simulink model "nominal_system"  (R2018a)
settings: Solver=ode8  StartTime=0.0  StopTime=10  FixedStep=.001  MaxStep=0.01  MinStep=.001  RelTol=1e-3
values from neighbouring files (symbols this model uses):
  a = 1.4    [Codefile.m]
  alpha1 = 0    [Codefile.m]
  Ap1 = 0    [Codefile.m]
  b = 1.7    [Codefile.m]
  beta1 = 0    [Codefile.m]
  c = 1.5    [Codefile.m]    (also in Quater_car.m = [700 1500 3000])
  Csfl = 1000    [Codefile.m]
  Csfr = 1000    [Codefile.m]
  Csrl = 1100    [Codefile.m]
  Csrr = 1100    [Codefile.m]
  d = 1.5    [Codefile.m]
  delay = (a+b)/v    (= 0.3875)    [Codefile.m]
  G = [ 0          0      0           0, ... (first row only)    [Codefile.m]
  gama1 = 0    [Codefile.m]
  Ixx = 460    [Codefile.m]
  Iyy = 2160    [Codefile.m]
  Ksfl = 35000    [Codefile.m]
  Ksfr = 35000    [Codefile.m]
  Ksrl = 38000    [Codefile.m]
  Ksrr = 38000    [Codefile.m]
  Kufl = 190000    [Codefile.m]
  Kufr = 190000    [Codefile.m]
  Kurl = 190000    [Codefile.m]
  Kurr = 190000    [Codefile.m]
  M = 1500    [Codefile.m]    (also in Quater_car.m = 117; half_car.m = 117)
  m = 59    [Codefile.m]    (also in Quater_car.m = 30)
  Ps1 = 0    [Codefile.m]
  tau1 = 1    [Codefile.m]
settings Model: Creator=Student  LastModifiedBy=Student
settings SolverCC: InitialStep=.001

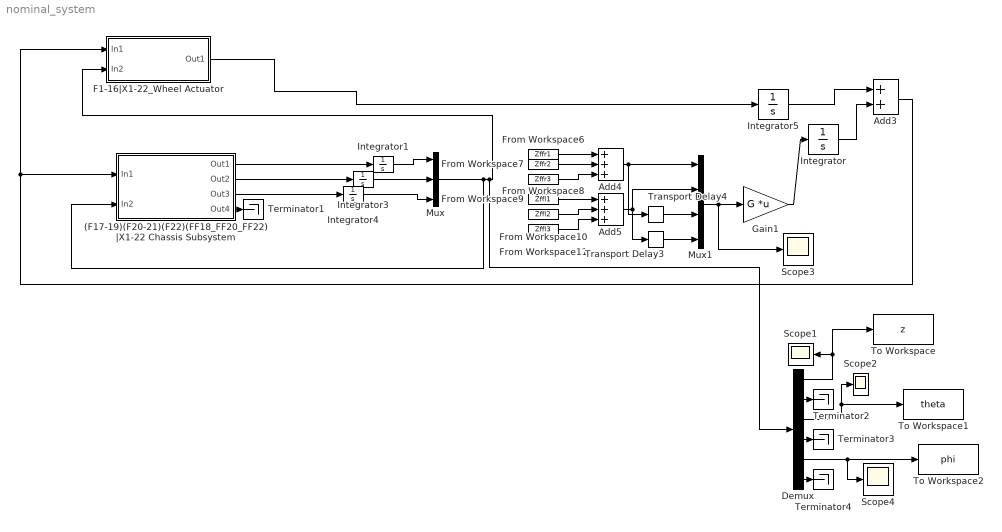
== system nominal_system ==
  "(F17-19)(F20-21)(F22)(FF18_FF20_FF22) |X1-22 Chassis Subsystem " : Subsystem  TreatAsAtomicUnit=on
  Add3 : Sum  Inputs=2
  Add4 : Sum  Inputs=3
  Add5 : Sum  Inputs=3
  Demux : Demux  Outputs=6
  "F1-16|X1-22_Wheel Actuator " : Subsystem  TreatAsAtomicUnit=on
  From Workspace10 : FromWorkspace  VariableName=Zffl2  SampleTime=0  Interpolate=off  OutputAfterFinalValue=Setting to zero
  From Workspace11 : FromWorkspace  VariableName=Zffl3  SampleTime=0  Interpolate=off  OutputAfterFinalValue=Setting to zero
  From Workspace6 : FromWorkspace  VariableName=Zffr1  SampleTime=0  Interpolate=off  OutputAfterFinalValue=Setting to zero
  From Workspace7 : FromWorkspace  VariableName=Zffr2  SampleTime=0  Interpolate=off  OutputAfterFinalValue=Setting to zero
  From Workspace8 : FromWorkspace  VariableName=Zffr3  SampleTime=0  Interpolate=off  OutputAfterFinalValue=Setting to zero
  From Workspace9 : FromWorkspace  VariableName=Zffl1  SampleTime=0  Interpolate=off  OutputAfterFinalValue=Setting to zero
  Gain1 : Gain  Gain=G  Multiplication=Matrix(K*u)
  Integrator{,1,3..5} (5 alike) : Integrator  AbsoluteTolerance=1e-4
  Mux : Mux  Inputs=3
  Mux1 : Mux
  Scope{1..4} (4 alike) : Scope
  Terminator{1..4} (4 alike) : Terminator
  To Workspace : ToWorkspace  VariableName=z  SaveFormat=Timeseries  SampleTime=-1
  To Workspace1 : ToWorkspace  VariableName=theta  SaveFormat=Timeseries  SampleTime=-1
  To Workspace2 : ToWorkspace  VariableName=phi  SaveFormat=Timeseries  SampleTime=-1
  Transport Delay3 : TransportDelay  DelayTime=delay
  Transport Delay4 : TransportDelay  DelayTime=delay
  wires:
  Demux/6 -> Terminator4/1
  Integrator4/1 -> Mux/3
  Demux/2 -> Terminator2/1
  Demux/3 -> Scope2/1, To Workspace1/1
  Integrator/1 -> Add3/2
  Integrator1/1 -> Mux/1
  Integrator3/1 -> Mux/2
  Integrator5/1 -> Add3/1
  "F1-16|X1-22_Wheel Actuator "/1(Out1) -> Integrator5/1
  "(F17-19)(F20-21)(F22)(FF18_FF20_FF22) |X1-22 Chassis Subsystem "/3(Out3) -> Integrator4/1
  Add3/1 -> "F1-16|X1-22_Wheel Actuator "/1(In1), "(F17-19)(F20-21)(F22)(FF18_FF20_FF22) |X1-22 Chassis Subsystem "/1(In1)
  Mux/1 -> "(F17-19)(F20-21)(F22)(FF18_FF20_FF22) |X1-22 Chassis Subsystem "/2(In2), Demux/1, "F1-16|X1-22_Wheel Actuator "/2(In2)
  Demux/4 -> Terminator3/1
  "(F17-19)(F20-21)(F22)(FF18_FF20_FF22) |X1-22 Chassis Subsystem "/2(Out2) -> Integrator3/1
  Gain1/1 -> Integrator/1
  "(F17-19)(F20-21)(F22)(FF18_FF20_FF22) |X1-22 Chassis Subsystem "/1(Out1) -> Integrator1/1
  Demux/5 -> To Workspace2/1, Scope4/1
  "(F17-19)(F20-21)(F22)(FF18_FF20_FF22) |X1-22 Chassis Subsystem "/4(Out4) -> Terminator1/1
  From Workspace7/1 -> Add4/2
  From Workspace10/1 -> Add5/2
  From Workspace11/1 -> Add5/3
  From Workspace9/1 -> Add5/1
  Add5/1 -> Mux1/2, Transport Delay3/1
  From Workspace6/1 -> Add4/1
  From Workspace8/1 -> Add4/3
  Mux1/1 -> Scope3/1, Gain1/1
  Add4/1 -> Mux1/1, Transport Delay4/1
  Transport Delay4/1 -> Mux1/3
  Transport Delay3/1 -> Mux1/4
  Demux/1 -> To Workspace/1, Scope1/1

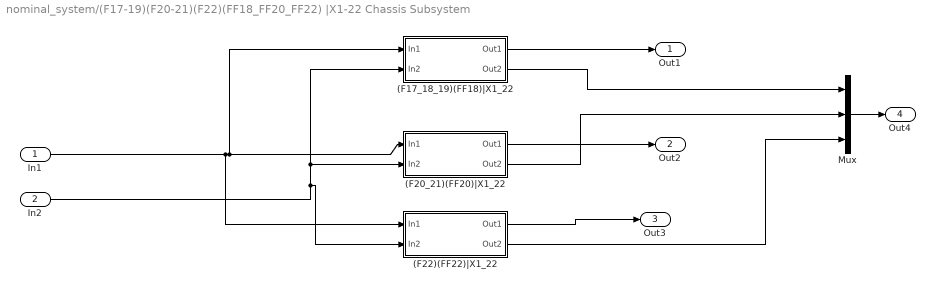
== system nominal_system/(F17-19)(F20-21)(F22)(FF18_FF20_FF22) |X1-22 Chassis Subsystem  ==
  In1 : Inport
  In2 : Inport  Port=2
  (F17_18_19)(FF18)|X1_22 : Subsystem  TreatAsAtomicUnit=on
  "(F20_21)(FF20)|X1_22 " : Subsystem  TreatAsAtomicUnit=on
  (F22)(FF22)|X1_22 : Subsystem  TreatAsAtomicUnit=on
  Mux : Mux  Inputs=3
  Out1 : Outport
  Out2 : Outport  Port=2
  Out3 : Outport  Port=3
  Out4 : Outport  Port=4
  wires:
  In1/1 -> (F17_18_19)(FF18)|X1_22/1(In1), "(F20_21)(FF20)|X1_22 "/1(In1), (F22)(FF22)|X1_22/1(In1)
  (F22)(FF22)|X1_22/1(Out1) -> Out3/1
  "(F20_21)(FF20)|X1_22 "/1(Out1) -> Out2/1
  (F17_18_19)(FF18)|X1_22/1(Out1) -> Out1/1
  (F17_18_19)(FF18)|X1_22/2(Out2) -> Mux/1
  "(F20_21)(FF20)|X1_22 "/2(Out2) -> Mux/2
  (F22)(FF22)|X1_22/2(Out2) -> Mux/3
  Mux/1 -> Out4/1
  In2/1 -> (F22)(FF22)|X1_22/2(In2), "(F20_21)(FF20)|X1_22 "/2(In2), (F17_18_19)(FF18)|X1_22/2(In2)

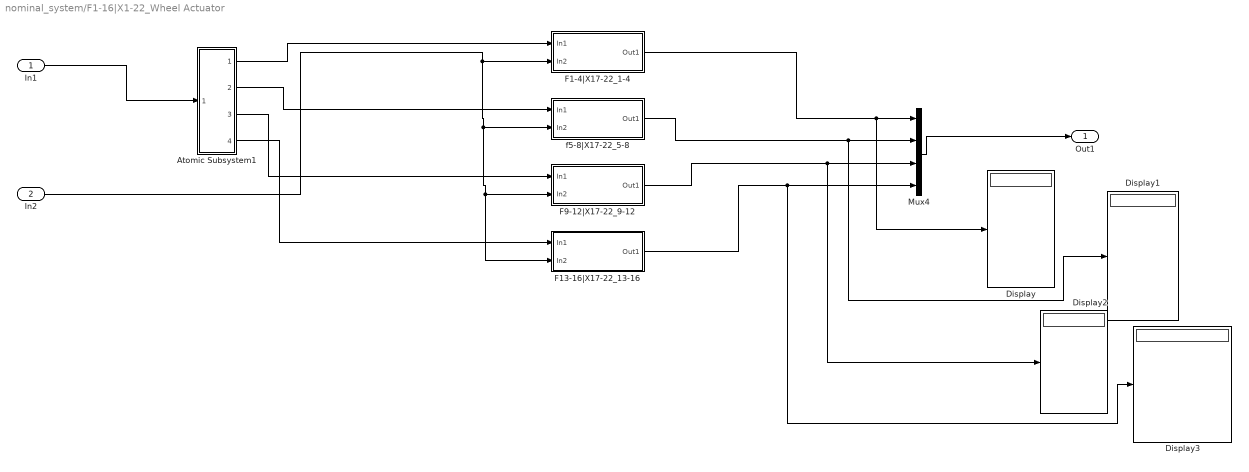
== system nominal_system/F1-16|X1-22_Wheel Actuator  ==
  In1 : Inport
  In2 : Inport  Port=2
  Atomic Subsystem1 : Subsystem  TreatAsAtomicUnit=on
  Display{,1..3} (4 alike) : Display
  F1-4|X17-22_1-4 : Subsystem  TreatAsAtomicUnit=on
  F13-16|X17-22_13-16 : Subsystem  TreatAsAtomicUnit=on
  F9-12|X17-22_9-12 : Subsystem  TreatAsAtomicUnit=on
  Mux4 : Mux
  f5-8|X17-22_5-8 : Subsystem  TreatAsAtomicUnit=on
  Out1 : Outport
  wires:
  In1/1 -> Atomic Subsystem1/1(In1)
  Mux4/1 -> Out1/1
  Atomic Subsystem1/1(Out1) -> F1-4|X17-22_1-4/1(In1)
  Atomic Subsystem1/2(Out2) -> f5-8|X17-22_5-8/1(In1)
  Atomic Subsystem1/3(Out3) -> F9-12|X17-22_9-12/1(In1)
  Atomic Subsystem1/4(Out4) -> F13-16|X17-22_13-16/1(In1)
  In2/1 -> F13-16|X17-22_13-16/2(In2), F9-12|X17-22_9-12/2(In2), f5-8|X17-22_5-8/2(In2), F1-4|X17-22_1-4/2(In2)
  F1-4|X17-22_1-4/1(Out1) -> Display/1, Mux4/1
  f5-8|X17-22_5-8/1(Out1) -> Display1/1, Mux4/2
  F9-12|X17-22_9-12/1(Out1) -> Display2/1, Mux4/3
  F13-16|X17-22_13-16/1(Out1) -> Display3/1, Mux4/4

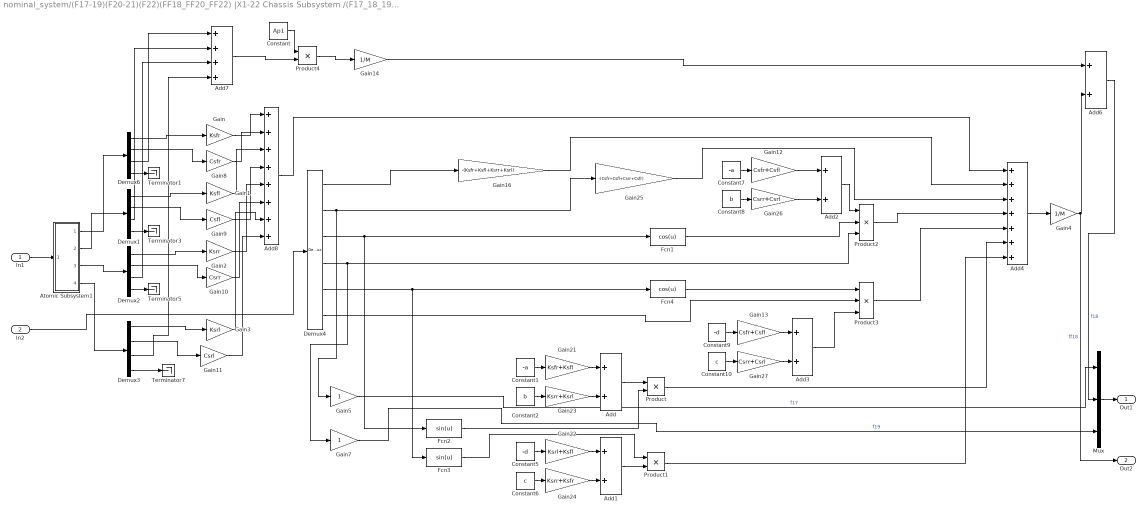
== system nominal_system/(F17-19)(F20-21)(F22)(FF18_FF20_FF22) |X1-22 Chassis Subsystem /(F17_18_19)(FF18)|X1_22 ==
  In1 : Inport
  In2 : Inport  Port=2
  Add{,1..3,6} (5 alike) : Sum
  Add4 : Sum  Inputs=+++++++
  Add7 : Sum  Inputs=++++
  Add8 : Sum  Inputs=++++++++
  Atomic Subsystem1 : Subsystem  TreatAsAtomicUnit=on
  Constant : Constant  Value=Ap1
  Constant1 : Constant  Value=-a
  Constant10 : Constant  Value=c
  Constant2 : Constant  Value=b
  Constant5 : Constant  Value=-d
  Constant6 : Constant  Value=c
  Constant7 : Constant  Value=-a
  Constant8 : Constant  Value=b
  Constant9 : Constant  Value=-d
  Demux{1..3,6} (4 alike) : Demux
  Demux4 : Demux  Outputs=6
  Fcn1 : Fcn  Expr=cos(u)
  Fcn2 : Fcn  Expr=sin(u)
  Fcn3 : Fcn  Expr=sin(u)
  Fcn4 : Fcn  Expr=cos(u)
  Gain : Gain  Gain=Ksfr
  Gain1 : Gain  Gain=Ksfl
  Gain10 : Gain  Gain=Csrr
  Gain11 : Gain  Gain=Csrl
  Gain12 : Gain  Gain=Csfr+Csfl
  Gain13 : Gain  Gain=Csfr+Csfl
  Gain14 : Gain  Gain=1/M
  Gain16 : Gain  Gain=-(Ksfr+Ksfl+Ksrr+Ksrl)
  Gain2 : Gain  Gain=Ksrr
  Gain21 : Gain  Gain=Ksfr+Ksfl
  Gain22 : Gain  Gain=Ksrl+Ksfl
  Gain23 : Gain  Gain=Ksrr+Ksrl
  Gain24 : Gain  Gain=Ksrr+Ksfr
  Gain25 : Gain  Gain=-(Csfr+Csfl+Csrr+Csfr)
  Gain26 : Gain  Gain=Csrr+Csrl
  Gain27 : Gain  Gain=Csrr+Csrl
  Gain3 : Gain  Gain=Ksrl
  Gain4 : Gain  Gain=1/M
  Gain5 : Gain
  Gain7 : Gain
  Gain8 : Gain  Gain=Csfr
  Gain9 : Gain  Gain=Csfl
  Mux : Mux  Inputs=3
  Product : Product
  Product1 : Product
  Product2 : Product  Inputs=3
  Product3 : Product  Inputs=3
  Product4 : Product
  Terminator{1,3,5,7} (4 alike) : Terminator
  Out1 : Outport
  Out2 : Outport  Port=2
  wires:
  Demux6/1 -> Gain/1
  Demux1/1 -> Gain1/1
  Demux2/1 -> Gain2/1
  Demux3/1 -> Gain3/1
  Demux4/1 -> Gain16/1
  Demux4/3 -> Fcn2/1, Fcn1/1
  Gain21/1 -> Add/1
  Constant1/1 -> Gain21/1
  Gain23/1 -> Add/2
  Constant2/1 -> Gain23/1
  Add/1 -> Product/1
  Fcn2/1 -> Product/2
  Demux4/5 -> Fcn3/1, Fcn4/1
  Gain22/1 -> Add1/1
  Gain24/1 -> Add1/2
  Constant5/1 -> Gain22/1
  Constant6/1 -> Gain24/1
  Add1/1 -> Product1/2
  Fcn3/1 -> Product1/1
  Demux4/2 -> Gain5/1, Gain25/1
  Demux4/4 -> Gain7/1, Product2/3
  Fcn1/1 -> Product2/2
  Gain12/1 -> Add2/1
  Constant7/1 -> Gain12/1
  Gain26/1 -> Add2/2
  Constant8/1 -> Gain26/1
  Add2/1 -> Product2/1
  Gain13/1 -> Add3/1
  Constant9/1 -> Gain13/1
  Gain27/1 -> Add3/2
  Constant10/1 -> Gain27/1
  Fcn4/1 -> Product3/1
  Demux4/6 -> Product3/2
  Add3/1 -> Product3/3
  Product/1 -> Add4/6
  Product1/1 -> Add4/7
  Add4/1 -> Gain4/1
  Gain14/1 -> Add6/1
  Gain4/1 -> Out2/1, Add6/2  "ff18"
  Add6/1 -> Mux/2  "f18"
  Gain5/1 -> Mux/1  "f17"
  Gain7/1 -> Mux/3  "f19"
  Demux6/2 -> Gain8/1
  Demux1/2 -> Gain9/1
  Demux2/2 -> Gain10/1
  Demux3/2 -> Gain11/1
  Gain/1 -> Add8/1
  Gain8/1 -> Add8/2
  Gain1/1 -> Add8/3
  Gain9/1 -> Add8/4
  Gain2/1 -> Add8/5
  Gain10/1 -> Add8/6
  Gain3/1 -> Add8/7
  Gain11/1 -> Add8/8
  Product3/1 -> Add4/5
  Product2/1 -> Add4/4
  Gain25/1 -> Add4/3
  Gain16/1 -> Add4/2
  Add8/1 -> Add4/1
  Demux6/3 -> Add7/1
  Demux6/4 -> Terminator1/1
  Demux1/3 -> Add7/2
  Demux1/4 -> Terminator3/1
  Demux2/3 -> Add7/3
  Demux2/4 -> Terminator5/1
  Demux3/3 -> Add7/4
  Demux3/4 -> Terminator7/1
  Mux/1 -> Out1/1
  Add7/1 -> Product4/2
  Constant/1 -> Product4/1
  Product4/1 -> Gain14/1
  In1/1 -> Atomic Subsystem1/1(In1)
  Atomic Subsystem1/1(Out1) -> Demux6/1
  Atomic Subsystem1/2(Out2) -> Demux1/1
  Atomic Subsystem1/3(Out3) -> Demux2/1
  Atomic Subsystem1/4(Out4) -> Demux3/1
  In2/1 -> Demux4/1

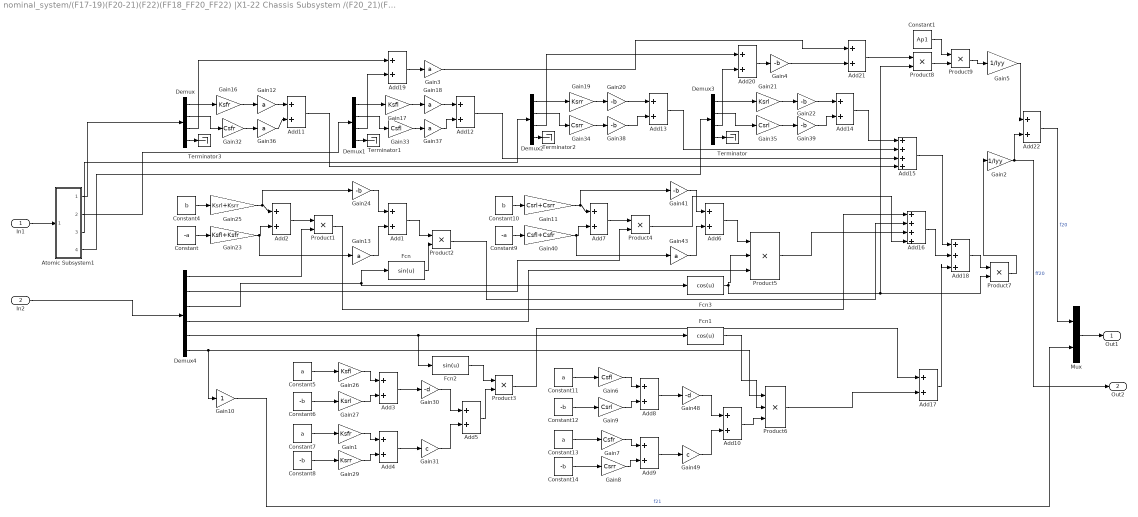
== system nominal_system/(F17-19)(F20-21)(F22)(FF18_FF20_FF22) |X1-22 Chassis Subsystem /(F20_21)(FF20)|X1_22  ==
  In1 : Inport
  In2 : Inport  Port=2
  Add{1..14,17,19..22} (19 alike) : Sum
  Add15 : Sum  Inputs=++++
  Add16 : Sum  Inputs=++++
  Add18 : Sum  Inputs=+++
  Atomic Subsystem1 : Subsystem  TreatAsAtomicUnit=on
  Constant : Constant  Value=-a
  Constant1 : Constant  Value=Ap1
  Constant10 : Constant  Value=b
  Constant{5,7,11,13} (4 alike) : Constant  Value=a
  Constant{6,8,12,14} (4 alike) : Constant  Value=-b
  Constant4 : Constant  Value=b
  Constant9 : Constant  Value=-a
  Demux{,1..3} (4 alike) : Demux
  Demux4 : Demux  Outputs=6
  Fcn : Fcn  Expr=sin(u)
  Fcn1 : Fcn  Expr=cos(u)
  Fcn2 : Fcn  Expr=sin(u)
  Fcn3 : Fcn  Expr=cos(u)
  Gain1 : Gain  Gain=Ksfr
  Gain10 : Gain
  Gain11 : Gain  Gain=Csrl+Csrr
  Gain{3,12..13,18,36..37,43} (7 alike) : Gain  Gain=a
  Gain16 : Gain  Gain=Ksfr
  Gain17 : Gain  Gain=Ksfl
  Gain19 : Gain  Gain=Ksrr
  Gain2 : Gain  Gain=1/Iyy
  Gain{4,20,22,24,38..39,41} (7 alike) : Gain  Gain=-b
  Gain21 : Gain  Gain=Ksrl
  Gain23 : Gain  Gain=Ksfl+Ksfr
  Gain25 : Gain  Gain=Ksrl+Ksrr
  Gain26 : Gain  Gain=Ksfl
  Gain27 : Gain  Gain=Ksrl
  Gain29 : Gain  Gain=Ksrr
  Gain30 : Gain  Gain=-d
  Gain31 : Gain  Gain=c
  Gain32 : Gain  Gain=Csfr
  Gain33 : Gain  Gain=Csfl
  Gain34 : Gain  Gain=Csrr
  Gain35 : Gain  Gain=Csrl
  Gain40 : Gain  Gain=Csfl+Csfr
  Gain48 : Gain  Gain=-d
  Gain49 : Gain  Gain=c
  Gain5 : Gain  Gain=1/Iyy
  Gain6 : Gain  Gain=Csfl
  Gain7 : Gain  Gain=Csfr
  Gain8 : Gain  Gain=Csrr
  Gain9 : Gain  Gain=Csrl
  Mux : Mux  Inputs=2
  Product{1..4,7..9} (7 alike) : Product
  Product5 : Product  Inputs=3
  Product6 : Product  Inputs=3
  Terminator{,1..3} (4 alike) : Terminator
  Out1 : Outport
  Out2 : Outport  Port=2
  wires:
  Demux/1 -> Gain16/1
  Gain16/1 -> Gain12/1
  Demux1/1 -> Gain17/1
  Gain17/1 -> Gain18/1
  Demux2/1 -> Gain19/1
  Gain19/1 -> Gain20/1
  Demux3/1 -> Gain21/1
  Gain21/1 -> Gain22/1
  Constant/1 -> Gain23/1
  Constant4/1 -> Gain25/1
  Gain23/1 -> Gain13/1, Add2/2
  Gain25/1 -> Gain24/1, Add2/1
  Add2/1 -> Product1/1
  Demux4/1 -> Product1/2
  Gain24/1 -> Add1/1
  Gain13/1 -> Add1/2
  Constant5/1 -> Gain26/1
  Constant6/1 -> Gain27/1
  Gain26/1 -> Add3/1
  Gain27/1 -> Add3/2
  Constant8/1 -> Gain29/1
  Constant7/1 -> Gain1/1
  Gain1/1 -> Add4/1
  Gain29/1 -> Add4/2
  Add3/1 -> Gain30/1
  Add4/1 -> Gain31/1
  Demux4/3 -> Fcn3/1, Fcn/1
  Add1/1 -> Product2/1
  Fcn/1 -> Product2/2
  Demux4/5 -> Fcn1/1, Fcn2/1
  Gain30/1 -> Add5/1
  Gain31/1 -> Add5/2
  Add5/1 -> Product3/2
  Fcn2/1 -> Product3/1
  Demux/2 -> Gain32/1
  Demux1/2 -> Gain33/1
  Demux2/2 -> Gain34/1
  Demux3/2 -> Gain35/1
  Gain32/1 -> Gain36/1
  Gain33/1 -> Gain37/1
  Gain34/1 -> Gain38/1
  Gain35/1 -> Gain39/1
  Constant10/1 -> Gain11/1
  Gain40/1 -> Gain43/1, Add7/2
  Gain11/1 -> Add7/1, Gain41/1
  Add7/1 -> Product4/1
  Demux4/2 -> Product4/2
  Gain41/1 -> Add6/1
  Gain43/1 -> Add6/2
  Add6/1 -> Product5/1
  Constant9/1 -> Gain40/1
  Fcn3/1 -> Product5/2, Product8/2, Product7/2
  Demux4/4 -> Product5/3
  Constant11/1 -> Gain6/1
  Constant12/1 -> Gain9/1
  Gain6/1 -> Add8/1
  Gain9/1 -> Add8/2
  Constant14/1 -> Gain8/1
  Constant13/1 -> Gain7/1
  Gain7/1 -> Add9/1
  Add8/1 -> Gain48/1
  Add9/1 -> Gain49/1
  Gain48/1 -> Add10/1
  Gain49/1 -> Add10/2
  Add10/1 -> Product6/3
  Fcn1/1 -> Product6/2
  Gain8/1 -> Add9/2
  Demux4/6 -> Gain10/1, Product6/1
  Gain12/1 -> Add11/1
  Gain36/1 -> Add11/2
  Gain18/1 -> Add12/1
  Gain37/1 -> Add12/2
  Gain20/1 -> Add13/1
  Gain38/1 -> Add13/2
  Gain22/1 -> Add14/1
  Gain39/1 -> Add14/2
  Add14/1 -> Add15/1
  Add13/1 -> Add15/2
  Add12/1 -> Add15/3
  Add11/1 -> Add15/4
  Product1/1 -> Add16/1
  Product2/1 -> Add16/2
  Product5/1 -> Add16/3
  Product4/1 -> Add16/4
  Product3/1 -> Add17/1
  Product6/1 -> Add17/2
  Add15/1 -> Add18/1
  Add17/1 -> Add18/3
  Add16/1 -> Add18/2
  Add18/1 -> Product7/1
  Product7/1 -> Gain2/1
  Demux/3 -> Add19/1
  Demux1/3 -> Add19/2
  Add19/1 -> Gain3/1
  Demux2/3 -> Add20/1
  Demux3/3 -> Add20/2
  Add20/1 -> Gain4/1
  Gain4/1 -> Add21/2
  Gain3/1 -> Add21/1
  Add21/1 -> Product8/1
  Gain5/1 -> Add22/1
  Gain2/1 -> Out2/1, Add22/2  "ff20"
  Gain10/1 -> Mux/2  "f21"
  Add22/1 -> Mux/1  "f20"
  Demux1/4 -> Terminator1/1
  Demux2/4 -> Terminator2/1
  Demux3/4 -> Terminator/1
  Demux/4 -> Terminator3/1
  In2/1 -> Demux4/1
  Atomic Subsystem1/1(Out1) -> Demux/1
  Atomic Subsystem1/2(Out2) -> Demux1/1
  Atomic Subsystem1/3(Out3) -> Demux2/1
  Atomic Subsystem1/4(Out4) -> Demux3/1
  Mux/1 -> Out1/1
  Product8/1 -> Product9/2
  Product9/1 -> Gain5/1
  Constant1/1 -> Product9/1
  In1/1 -> Atomic Subsystem1/1(In1)

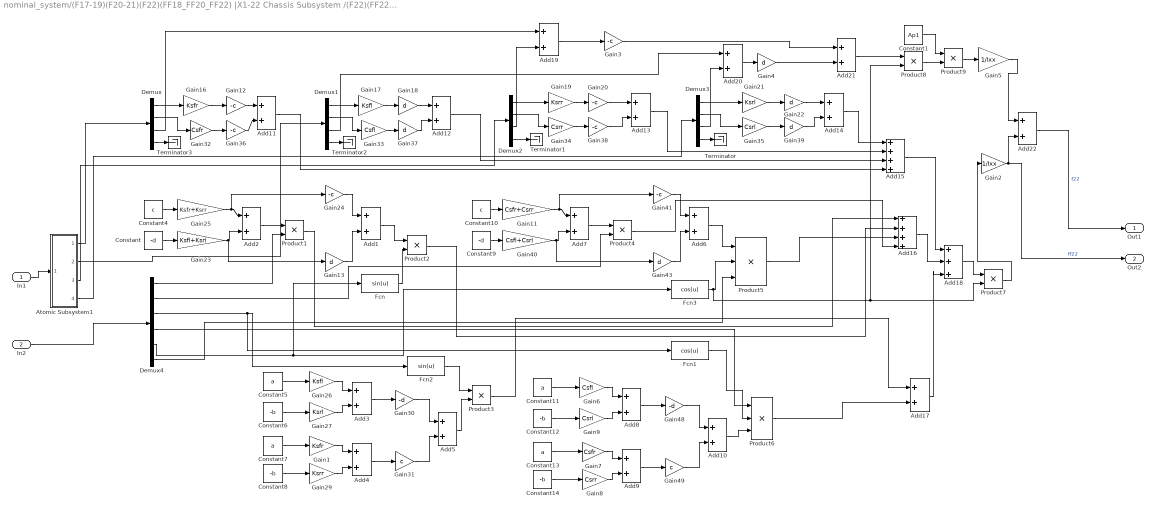
== system nominal_system/(F17-19)(F20-21)(F22)(FF18_FF20_FF22) |X1-22 Chassis Subsystem /(F22)(FF22)|X1_22 ==
  In1 : Inport
  In2 : Inport  Port=2
  Add{1..14,17,19..22} (19 alike) : Sum
  Add15 : Sum  Inputs=++++
  Add16 : Sum  Inputs=++++
  Add18 : Sum  Inputs=+++
  Atomic Subsystem1 : Subsystem  TreatAsAtomicUnit=on
  Constant : Constant  Value=-d
  Constant1 : Constant  Value=Ap1
  Constant10 : Constant  Value=c
  Constant{5,7,11,13} (4 alike) : Constant  Value=a
  Constant{6,8,12,14} (4 alike) : Constant  Value=-b
  Constant4 : Constant  Value=c
  Constant9 : Constant  Value=-d
  Demux{,1..3} (4 alike) : Demux
  Demux4 : Demux  Outputs=6
  Fcn : Fcn  Expr=sin(u)
  Fcn1 : Fcn  Expr=cos(u)
  Fcn2 : Fcn  Expr=sin(u)
  Fcn3 : Fcn  Expr=cos(u)
  Gain1 : Gain  Gain=Ksfr
  Gain11 : Gain  Gain=Csfr+Csrr
  Gain{3,12,20,24,36,38,41} (7 alike) : Gain  Gain=-c
  Gain{4,13,18,22,37,39,43} (7 alike) : Gain  Gain=d
  Gain16 : Gain  Gain=Ksfr
  Gain17 : Gain  Gain=Ksfl
  Gain19 : Gain  Gain=Ksrr
  Gain2 : Gain  Gain=1/Ixx
  Gain21 : Gain  Gain=Ksrl
  Gain23 : Gain  Gain=Ksfl+Ksrl
  Gain25 : Gain  Gain=Ksfr+Ksrr
  Gain26 : Gain  Gain=Ksfl
  Gain27 : Gain  Gain=Ksrl
  Gain29 : Gain  Gain=Ksrr
  Gain30 : Gain  Gain=-d
  Gain31 : Gain  Gain=c
  Gain32 : Gain  Gain=Csfr
  Gain33 : Gain  Gain=Csfl
  Gain34 : Gain  Gain=Csrr
  Gain35 : Gain  Gain=Csrl
  Gain40 : Gain  Gain=Csfl+Csrl
  Gain48 : Gain  Gain=-d
  Gain49 : Gain  Gain=c
  Gain5 : Gain  Gain=1/Ixx
  Gain6 : Gain  Gain=Csfl
  Gain7 : Gain  Gain=Csfr
  Gain8 : Gain  Gain=Csrr
  Gain9 : Gain  Gain=Csrl
  Product{1..4,7..9} (7 alike) : Product
  Product5 : Product  Inputs=3
  Product6 : Product  Inputs=3
  Terminator{,1..3} (4 alike) : Terminator
  Out1 : Outport
  Out2 : Outport  Port=2
  wires:
  Demux/1 -> Gain16/1
  Gain16/1 -> Gain12/1
  Demux1/1 -> Gain17/1
  Gain17/1 -> Gain18/1
  Demux2/1 -> Gain19/1
  Gain19/1 -> Gain20/1
  Demux3/1 -> Gain21/1
  Gain21/1 -> Gain22/1
  Constant/1 -> Gain23/1
  Constant4/1 -> Gain25/1
  Gain23/1 -> Gain13/1, Add2/2
  Gain25/1 -> Gain24/1, Add2/1
  Add2/1 -> Product1/1
  Demux4/1 -> Product1/2
  Gain24/1 -> Add1/1
  Gain13/1 -> Add1/2
  Constant5/1 -> Gain26/1
  Constant6/1 -> Gain27/1
  Gain26/1 -> Add3/1
  Gain27/1 -> Add3/2
  Constant8/1 -> Gain29/1
  Constant7/1 -> Gain1/1
  Gain1/1 -> Add4/1
  Gain29/1 -> Add4/2
  Add3/1 -> Gain30/1
  Add4/1 -> Gain31/1
  Demux4/3 -> Fcn1/1, Fcn2/1
  Add1/1 -> Product2/1
  Fcn/1 -> Product2/2
  Demux4/5 -> Fcn/1, Fcn3/1
  Gain30/1 -> Add5/1
  Gain31/1 -> Add5/2
  Add5/1 -> Product3/2
  Fcn2/1 -> Product3/1
  Demux/2 -> Gain32/1
  Demux1/2 -> Gain33/1
  Demux2/2 -> Gain34/1
  Demux3/2 -> Gain35/1
  Gain32/1 -> Gain36/1
  Gain33/1 -> Gain37/1
  Gain34/1 -> Gain38/1
  Gain35/1 -> Gain39/1
  Constant10/1 -> Gain11/1
  Gain40/1 -> Gain43/1, Add7/2
  Gain11/1 -> Add7/1, Gain41/1
  Add7/1 -> Product4/1
  Demux4/2 -> Product4/2
  Gain41/1 -> Add6/1
  Gain43/1 -> Add6/2
  Add6/1 -> Product5/1
  Constant9/1 -> Gain40/1
  Fcn3/1 -> Product8/2, Product7/2, Product5/2
  Constant11/1 -> Gain6/1
  Constant12/1 -> Gain9/1
  Gain6/1 -> Add8/1
  Gain9/1 -> Add8/2
  Constant14/1 -> Gain8/1
  Constant13/1 -> Gain7/1
  Gain7/1 -> Add9/1
  Add8/1 -> Gain48/1
  Add9/1 -> Gain49/1
  Gain48/1 -> Add10/1
  Gain49/1 -> Add10/2
  Add10/1 -> Product6/3
  Fcn1/1 -> Product6/2
  Gain8/1 -> Add9/2
  Demux4/6 -> Product5/3
  Gain12/1 -> Add11/1
  Gain36/1 -> Add11/2
  Gain18/1 -> Add12/1
  Gain37/1 -> Add12/2
  Gain20/1 -> Add13/1
  Gain38/1 -> Add13/2
  Gain22/1 -> Add14/1
  Gain39/1 -> Add14/2
  Add14/1 -> Add15/1
  Add13/1 -> Add15/2
  Add12/1 -> Add15/3
  Add11/1 -> Add15/4
  Product1/1 -> Add16/1
  Product2/1 -> Add16/2
  Product5/1 -> Add16/3
  Product4/1 -> Add16/4
  Product3/1 -> Add17/1
  Product6/1 -> Add17/2
  Add15/1 -> Add18/1
  Add17/1 -> Add18/3
  Add16/1 -> Add18/2
  Add18/1 -> Product7/1
  Product7/1 -> Gain2/1
  Demux/3 -> Add19/1
  Add19/1 -> Gain3/1
  Add20/1 -> Gain4/1
  Gain4/1 -> Add21/2
  Gain3/1 -> Add21/1
  Add21/1 -> Product8/1
  Gain5/1 -> Add22/1
  Gain2/1 -> Out2/1, Add22/2  "ff22"
  Add22/1 -> Out1/1  "f22"
  Demux4/4 -> Product6/1
  Demux2/3 -> Add19/2
  Demux1/3 -> Add20/1
  Demux3/3 -> Add20/2
  In2/1 -> Demux4/1
  Atomic Subsystem1/1(Out1) -> Demux/1
  Atomic Subsystem1/2(Out2) -> Demux1/1
  Atomic Subsystem1/3(Out3) -> Demux2/1
  Atomic Subsystem1/4(Out4) -> Demux3/1
  Demux3/4 -> Terminator/1
  Demux2/4 -> Terminator1/1
  Demux1/4 -> Terminator2/1
  Demux/4 -> Terminator3/1
  In1/1 -> Atomic Subsystem1/1(In1)
  Product9/1 -> Gain5/1
  Product8/1 -> Product9/2
  Constant1/1 -> Product9/1

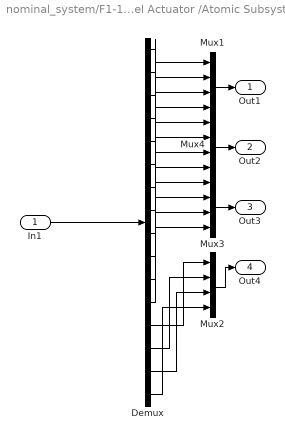
== system nominal_system/F1-16|X1-22_Wheel Actuator /Atomic Subsystem1 ==
  In1 : Inport
  Demux : Demux  Outputs=16
  Mux{1..4} (4 alike) : Mux
  Out1 : Outport
  Out2 : Outport  Port=2
  Out3 : Outport  Port=3
  Out4 : Outport  Port=4
  wires:
  In1/1 -> Demux/1
  Demux/16 -> Mux2/4
  Demux/15 -> Mux2/3
  Demux/14 -> Mux2/2
  Demux/13 -> Mux2/1
  Demux/12 -> Mux3/4
  Demux/11 -> Mux3/3
  Demux/10 -> Mux3/2
  Demux/9 -> Mux3/1
  Demux/8 -> Mux4/4
  Demux/7 -> Mux4/3
  Demux/6 -> Mux4/2
  Demux/5 -> Mux4/1
  Demux/4 -> Mux1/4
  Demux/3 -> Mux1/3
  Demux/2 -> Mux1/2
  Demux/1 -> Mux1/1
  Mux1/1 -> Out1/1
  Mux4/1 -> Out2/1
  Mux3/1 -> Out3/1
  Mux2/1 -> Out4/1

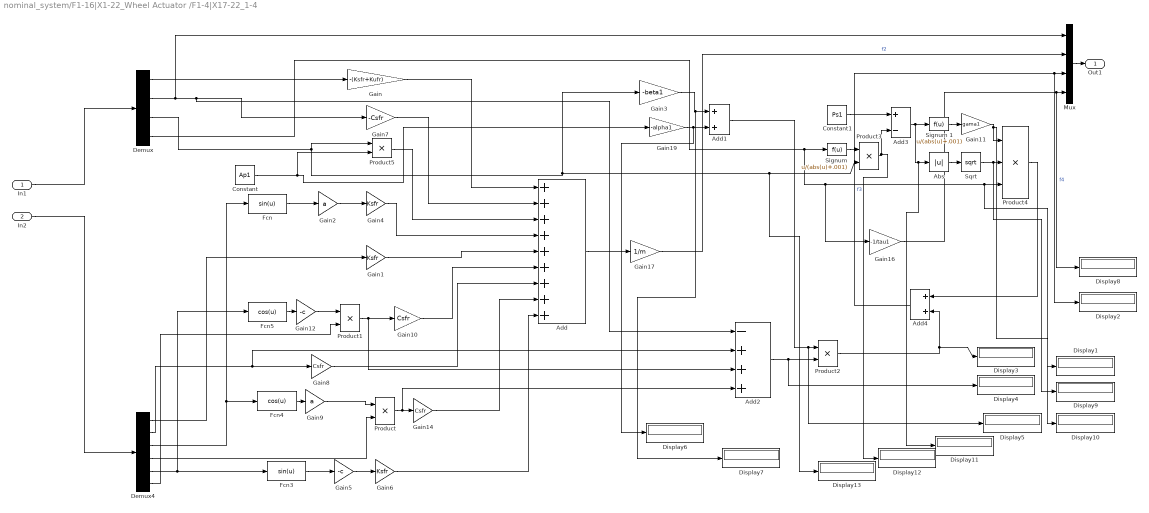
== system nominal_system/F1-16|X1-22_Wheel Actuator /F1-4|X17-22_1-4 ==
  In1 : Inport
  In2 : Inport  Port=2
  Abs : Abs
  Add : Sum  Inputs=+++++++++
  Add1 : Sum
  Add2 : Sum  Inputs=-+++
  Add3 : Sum  Inputs=+-
  Add4 : Sum
  Constant : Constant  Value=Ap1
  Constant1 : Constant  Value=Ps1
  Demux : Demux
  Demux4 : Demux  Outputs=6
  Display{1..13} (13 alike) : Display
  Fcn : Fcn  Expr=sin(u)
  Fcn3 : Fcn  Expr=sin(u)
  Fcn4 : Fcn  Expr=cos(u)
  Fcn5 : Fcn  Expr=cos(u)
  Gain : Gain  Gain=-(Ksfr+Kufr)
  Gain1 : Gain  Gain=Ksfr
  Gain10 : Gain  Gain=Csfr
  Gain11 : Gain  Gain=gama1
  Gain12 : Gain  Gain=-c
  Gain14 : Gain  Gain=Csfr
  Gain16 : Gain  Gain=-1/tau1
  Gain17 : Gain  Gain=1/m
  Gain19 : Gain  Gain=-alpha1
  Gain2 : Gain  Gain=a
  Gain3 : Gain  Gain=-beta1
  Gain4 : Gain  Gain=Ksfr
  Gain5 : Gain  Gain=-c
  Gain6 : Gain  Gain=Ksfr
  Gain7 : Gain  Gain=-Csfr
  Gain8 : Gain  Gain=Csfr
  Gain9 : Gain  Gain=a
  Mux : Mux
  Product{,1..3,5} (5 alike) : Product
  Product4 : Product  Inputs=3
  "Signum " : Fcn  Expr=u/(abs(u)+.001)
  Signum 1 : Fcn  Expr=u/(abs(u)+.001)
  Sqrt : Sqrt  SaturateOnIntegerOverflow=on
  Out1 : Outport
  wires:
  Demux4/1 -> Gain1/1
  Demux4/3 -> Fcn/1, Fcn4/1
  Fcn/1 -> Gain2/1
  Gain2/1 -> Gain4/1
  Demux4/5 -> Fcn5/1, Fcn3/1
  Fcn3/1 -> Gain5/1
  Gain5/1 -> Gain6/1
  Demux/2 -> Mux/1, Add2/1, Gain7/1
  Demux4/2 -> Add2/2, Gain8/1
  Fcn4/1 -> Gain9/1
  Gain9/1 -> Product/1
  Demux4/4 -> Product/2
  Fcn5/1 -> Gain12/1
  Demux4/6 -> Product1/2
  Gain12/1 -> Product1/1
  Demux/3 -> Product5/1, Gain3/1, Display13/1, Product3/2
  Gain/1 -> Add/1
  Gain7/1 -> Add/2
  Gain4/1 -> Add/4
  Gain1/1 -> Add/5
  Product1/1 -> Add2/3, Gain10/1
  Gain8/1 -> Add/7
  Product/1 -> Add2/4, Gain14/1
  Gain6/1 -> Add/9
  Gain3/1 -> Display7/1, Add1/1
  Gain19/1 -> Display6/1, Add1/2
  Gain14/1 -> Add/8
  Gain10/1 -> Add/6
  Add2/1 -> Display4/1, Product2/2
  Add1/1 -> Display5/1, Product2/1
  Demux/4 -> "Signum "/1, Gain16/1, Product4/3, Display10/1
  "Signum "/1 -> Product3/1
  Constant1/1 -> Add3/1
  Product3/1 -> Display12/1, Add3/2
  Signum 1/1 -> Gain11/1
  Abs/1 -> Sqrt/1
  Gain11/1 -> Display1/1, Product4/1
  Sqrt/1 -> Display9/1, Product4/2
  Product2/1 -> Display3/1, Add4/2
  Add/1 -> Gain17/1
  Gain17/1 -> Mux/2  "f2"
  Product4/1 -> Add4/1
  Add4/1 -> Display2/1, Mux/3  "f3"
  Gain16/1 -> Display8/1, Mux/4  "f4"
  Mux/1 -> Out1/1
  In1/1 -> Demux/1
  In2/1 -> Demux4/1
  Constant/1 -> Product5/2, Gain19/1
  Product5/1 -> Add/3
  Demux/1 -> Gain/1
  Add3/1 -> Signum 1/1, Display11/1, Abs/1

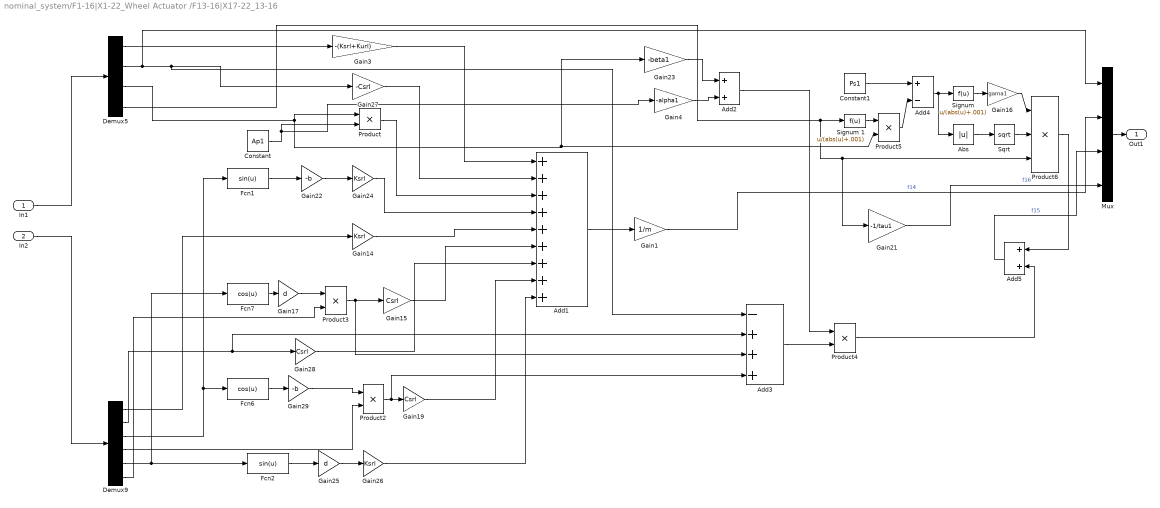
== system nominal_system/F1-16|X1-22_Wheel Actuator /F13-16|X17-22_13-16 ==
  In1 : Inport
  In2 : Inport  Port=2
  Abs : Abs
  Add1 : Sum  Inputs=+++++++++
  Add2 : Sum
  Add3 : Sum  Inputs=-+++
  Add4 : Sum  Inputs=+-
  Add5 : Sum
  Constant : Constant  Value=Ap1
  Constant1 : Constant  Value=Ps1
  Demux5 : Demux
  Demux9 : Demux  Outputs=6
  Fcn1 : Fcn  Expr=sin(u)
  Fcn2 : Fcn  Expr=sin(u)
  Fcn6 : Fcn  Expr=cos(u)
  Fcn7 : Fcn  Expr=cos(u)
  Gain1 : Gain  Gain=1/m
  Gain14 : Gain  Gain=Ksrl
  Gain15 : Gain  Gain=Csrl
  Gain16 : Gain  Gain=gama1
  Gain17 : Gain  Gain=d
  Gain19 : Gain  Gain=Csrl
  Gain21 : Gain  Gain=-1/tau1
  Gain22 : Gain  Gain=-b
  Gain23 : Gain  Gain=-beta1
  Gain24 : Gain  Gain=Ksrl
  Gain25 : Gain  Gain=d
  Gain26 : Gain  Gain=Ksrl
  Gain27 : Gain  Gain=-Csrl
  Gain28 : Gain  Gain=Csrl
  Gain29 : Gain  Gain=-b
  Gain3 : Gain  Gain=-(Ksrl+Kurl)
  Gain4 : Gain  Gain=-alpha1
  Mux : Mux
  Product{,2..5} (5 alike) : Product
  Product6 : Product  Inputs=3
  "Signum " : Fcn  Expr=u/(abs(u)+.001)
  Signum 1 : Fcn  Expr=u/(abs(u)+.001)
  Sqrt : Sqrt  SaturateOnIntegerOverflow=on
  Out1 : Outport
  wires:
  Demux5/1 -> Gain3/1
  Demux9/1 -> Gain14/1
  Demux9/3 -> Fcn1/1, Fcn6/1
  Fcn1/1 -> Gain22/1
  Gain22/1 -> Gain24/1
  Demux9/5 -> Fcn7/1, Fcn2/1
  Fcn2/1 -> Gain25/1
  Gain25/1 -> Gain26/1
  Demux9/2 -> Add3/2, Gain28/1
  Fcn6/1 -> Gain29/1
  Gain29/1 -> Product2/1
  Demux9/4 -> Product2/2
  Fcn7/1 -> Gain17/1
  Demux9/6 -> Product3/2
  Gain17/1 -> Product3/1
  Demux5/3 -> Product/1, Gain23/1, Product5/2
  Gain3/1 -> Add1/1
  Gain27/1 -> Add1/2
  Product/1 -> Add1/3
  Gain24/1 -> Add1/4
  Gain14/1 -> Add1/5
  Product3/1 -> Add3/3, Gain15/1
  Gain28/1 -> Add1/7
  Product2/1 -> Add3/4, Gain19/1
  Gain26/1 -> Add1/9
  Gain23/1 -> Add2/1
  Gain4/1 -> Add2/2
  Gain19/1 -> Add1/8
  Gain15/1 -> Add1/6
  Add3/1 -> Product4/2
  Add2/1 -> Product4/1
  Demux5/4 -> Signum 1/1, Gain21/1, Product6/3
  Signum 1/1 -> Product5/1
  Constant1/1 -> Add4/1
  Product5/1 -> Add4/2
  Add4/1 -> "Signum "/1, Abs/1
  "Signum "/1 -> Gain16/1
  Abs/1 -> Sqrt/1
  Gain16/1 -> Product6/1
  Sqrt/1 -> Product6/2
  Product4/1 -> Add5/2
  Add1/1 -> Gain1/1
  Gain1/1 -> Mux/2  "f14"
  Product6/1 -> Add5/1
  Add5/1 -> Mux/3  "f15"
  Gain21/1 -> Mux/4  "f16"
  Demux5/2 -> Mux/1, Add3/1, Gain27/1
  Mux/1 -> Out1/1
  In1/1 -> Demux5/1
  In2/1 -> Demux9/1
  Constant/1 -> Gain4/1, Product/2

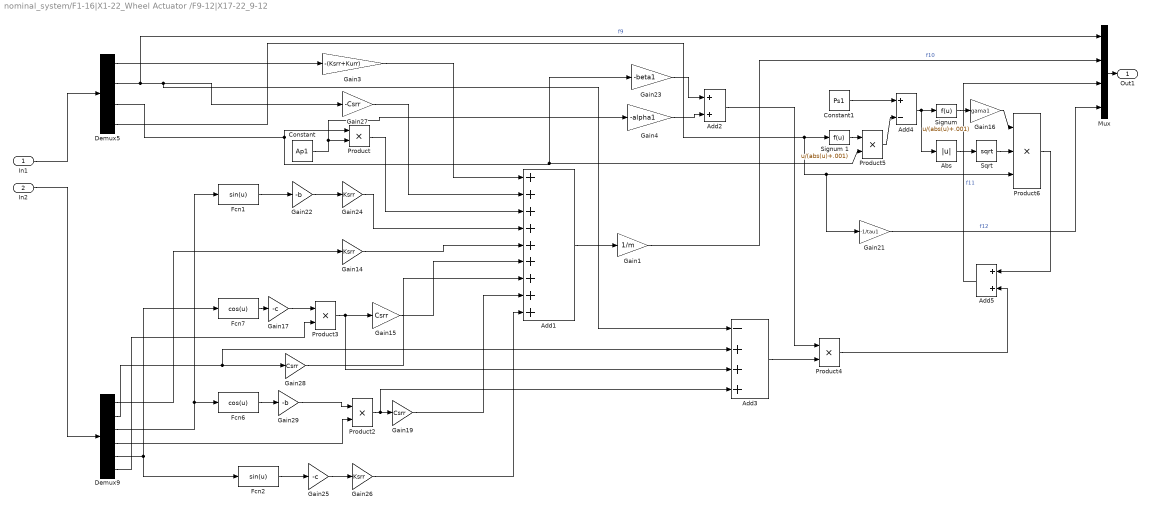
== system nominal_system/F1-16|X1-22_Wheel Actuator /F9-12|X17-22_9-12 ==
  In1 : Inport
  In2 : Inport  Port=2
  Abs : Abs
  Add1 : Sum  Inputs=+++++++++
  Add2 : Sum
  Add3 : Sum  Inputs=-+++
  Add4 : Sum  Inputs=+-
  Add5 : Sum
  Constant : Constant  Value=Ap1
  Constant1 : Constant  Value=Ps1
  Demux5 : Demux
  Demux9 : Demux  Outputs=6
  Fcn1 : Fcn  Expr=sin(u)
  Fcn2 : Fcn  Expr=sin(u)
  Fcn6 : Fcn  Expr=cos(u)
  Fcn7 : Fcn  Expr=cos(u)
  Gain1 : Gain  Gain=1/m
  Gain14 : Gain  Gain=Ksrr
  Gain15 : Gain  Gain=Csrr
  Gain16 : Gain  Gain=gama1
  Gain17 : Gain  Gain=-c
  Gain19 : Gain  Gain=Csrr
  Gain21 : Gain  Gain=-1/tau1
  Gain22 : Gain  Gain=-b
  Gain23 : Gain  Gain=-beta1
  Gain24 : Gain  Gain=Ksrr
  Gain25 : Gain  Gain=-c
  Gain26 : Gain  Gain=Ksrr
  Gain27 : Gain  Gain=-Csrr
  Gain28 : Gain  Gain=Csrr
  Gain29 : Gain  Gain=-b
  Gain3 : Gain  Gain=-(Ksrr+Kurr)
  Gain4 : Gain  Gain=-alpha1
  Mux : Mux
  Product{,2..5} (5 alike) : Product
  Product6 : Product  Inputs=3
  "Signum " : Fcn  Expr=u/(abs(u)+.001)
  Signum 1 : Fcn  Expr=u/(abs(u)+.001)
  Sqrt : Sqrt  SaturateOnIntegerOverflow=on
  Out1 : Outport
  wires:
  Demux5/1 -> Gain3/1
  Demux9/1 -> Gain14/1
  Demux9/3 -> Fcn1/1, Fcn6/1
  Fcn1/1 -> Gain22/1
  Gain22/1 -> Gain24/1
  Demux9/5 -> Fcn2/1, Fcn7/1
  Fcn2/1 -> Gain25/1
  Gain25/1 -> Gain26/1
  Demux9/2 -> Add3/2, Gain28/1
  Fcn6/1 -> Gain29/1
  Gain29/1 -> Product2/1
  Demux9/4 -> Product2/2
  Fcn7/1 -> Gain17/1
  Demux9/6 -> Product3/2
  Gain17/1 -> Product3/1
  Demux5/3 -> Product/1, Gain23/1, Product5/2
  Gain3/1 -> Add1/1
  Gain27/1 -> Add1/2
  Product/1 -> Add1/3
  Gain24/1 -> Add1/4
  Gain14/1 -> Add1/5
  Product3/1 -> Add3/3, Gain15/1
  Gain28/1 -> Add1/7
  Product2/1 -> Add3/4, Gain19/1
  Gain26/1 -> Add1/9
  Gain23/1 -> Add2/1
  Gain4/1 -> Add2/2
  Gain19/1 -> Add1/8
  Gain15/1 -> Add1/6
  Add3/1 -> Product4/2
  Add2/1 -> Product4/1
  Demux5/4 -> Signum 1/1, Gain21/1, Product6/3
  Signum 1/1 -> Product5/1
  Constant1/1 -> Add4/1
  Product5/1 -> Add4/2
  Add4/1 -> "Signum "/1, Abs/1
  "Signum "/1 -> Gain16/1
  Abs/1 -> Sqrt/1
  Gain16/1 -> Product6/1
  Sqrt/1 -> Product6/2
  Product4/1 -> Add5/2
  Add1/1 -> Gain1/1
  Demux5/2 -> Mux/1, Add3/1, Gain27/1  "f9"
  Gain1/1 -> Mux/2  "f10"
  Product6/1 -> Add5/1
  Add5/1 -> Mux/3  "f11"
  Gain21/1 -> Mux/4  "f12"
  Mux/1 -> Out1/1
  In1/1 -> Demux5/1
  In2/1 -> Demux9/1
  Constant/1 -> Product/2, Gain4/1

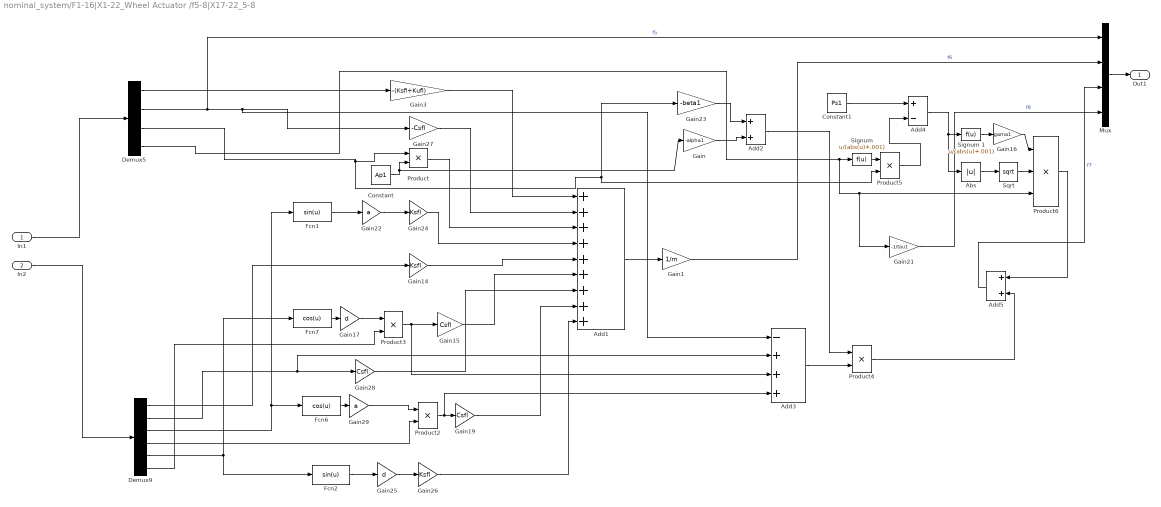
== system nominal_system/F1-16|X1-22_Wheel Actuator /f5-8|X17-22_5-8 ==
  In1 : Inport
  In2 : Inport  Port=2
  Abs : Abs
  Add1 : Sum  Inputs=+++++++++
  Add2 : Sum
  Add3 : Sum  Inputs=-+++
  Add4 : Sum  Inputs=+-
  Add5 : Sum
  Constant : Constant  Value=Ap1
  Constant1 : Constant  Value=Ps1
  Demux5 : Demux
  Demux9 : Demux  Outputs=6
  Fcn1 : Fcn  Expr=sin(u)
  Fcn2 : Fcn  Expr=sin(u)
  Fcn6 : Fcn  Expr=cos(u)
  Fcn7 : Fcn  Expr=cos(u)
  Gain : Gain  Gain=-alpha1
  Gain1 : Gain  Gain=1/m
  Gain14 : Gain  Gain=Ksfl
  Gain15 : Gain  Gain=Csfl
  Gain16 : Gain  Gain=gama1
  Gain17 : Gain  Gain=d
  Gain19 : Gain  Gain=Csfl
  Gain21 : Gain  Gain=-1/tau1
  Gain22 : Gain  Gain=a
  Gain23 : Gain  Gain=-beta1
  Gain24 : Gain  Gain=Ksfl
  Gain25 : Gain  Gain=d
  Gain26 : Gain  Gain=Ksfl
  Gain27 : Gain  Gain=-Csfl
  Gain28 : Gain  Gain=Csfl
  Gain29 : Gain  Gain=a
  Gain3 : Gain  Gain=-(Ksfl+Kufl)
  Mux : Mux
  Product{,2..5} (5 alike) : Product
  Product6 : Product  Inputs=3
  "Signum " : Fcn  Expr=u/(abs(u)+.001)
  Signum 1 : Fcn  Expr=u/(abs(u)+.001)
  Sqrt : Sqrt  SaturateOnIntegerOverflow=on
  Out1 : Outport
  wires:
  Demux5/1 -> Gain3/1
  Demux9/1 -> Gain14/1
  Demux9/3 -> Fcn1/1, Fcn6/1
  Fcn1/1 -> Gain22/1
  Gain22/1 -> Gain24/1
  Demux9/5 -> Fcn2/1, Fcn7/1
  Fcn2/1 -> Gain25/1
  Gain25/1 -> Gain26/1
  Demux9/2 -> Add3/2, Gain28/1
  Fcn6/1 -> Gain29/1
  Gain29/1 -> Product2/1
  Demux9/4 -> Product2/2
  Fcn7/1 -> Gain17/1
  Demux9/6 -> Product3/2
  Gain17/1 -> Product3/1
  Demux5/3 -> Product/1, Product5/2, Gain23/1
  Gain3/1 -> Add1/1
  Gain27/1 -> Add1/2
  Product/1 -> Add1/3
  Gain24/1 -> Add1/4
  Gain14/1 -> Add1/5
  Product3/1 -> Add3/3, Gain15/1
  Gain28/1 -> Add1/7
  Product2/1 -> Add3/4, Gain19/1
  Gain26/1 -> Add1/9
  Gain23/1 -> Add2/1
  Gain/1 -> Add2/2
  Gain19/1 -> Add1/8
  Gain15/1 -> Add1/6
  Add3/1 -> Product4/2
  Add2/1 -> Product4/1
  Demux5/4 -> "Signum "/1, Gain21/1, Product6/3
  "Signum "/1 -> Product5/1
  Constant1/1 -> Add4/1
  Product5/1 -> Add4/2
  Add4/1 -> Signum 1/1, Abs/1
  Signum 1/1 -> Gain16/1
  Abs/1 -> Sqrt/1
  Gain16/1 -> Product6/1
  Sqrt/1 -> Product6/2
  Product4/1 -> Add5/2
  Add1/1 -> Gain1/1
  Demux5/2 -> Mux/1, Add3/1, Gain27/1  "f5"
  Gain1/1 -> Mux/2  "f6"
  Product6/1 -> Add5/1
  Add5/1 -> Mux/3  "f7"
  Gain21/1 -> Mux/4  "f8"
  Mux/1 -> Out1/1
  In1/1 -> Demux5/1
  In2/1 -> Demux9/1
  Constant/1 -> Gain/1, Product/2

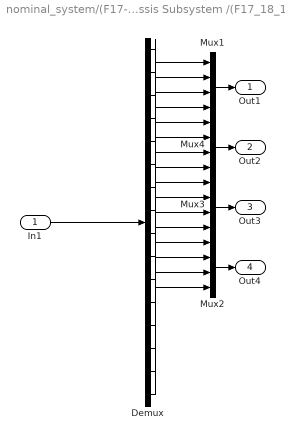
== system nominal_system/(F17-19)(F20-21)(F22)(FF18_FF20_FF22) |X1-22 Chassis Subsystem /(F17_18_19)(FF18)|X1_22/Atomic Subsystem1 ==
  In1 : Inport
  Demux : Demux  Outputs=16
  Mux{1..4} (4 alike) : Mux
  Out1 : Outport
  Out2 : Outport  Port=2
  Out3 : Outport  Port=3
  Out4 : Outport  Port=4
  wires:
  In1/1 -> Demux/1
  Demux/16 -> Mux2/4
  Demux/15 -> Mux2/3
  Demux/14 -> Mux2/2
  Demux/13 -> Mux2/1
  Demux/12 -> Mux3/4
  Demux/11 -> Mux3/3
  Demux/10 -> Mux3/2
  Demux/9 -> Mux3/1
  Demux/8 -> Mux4/4
  Demux/7 -> Mux4/3
  Demux/6 -> Mux4/2
  Demux/5 -> Mux4/1
  Demux/4 -> Mux1/4
  Demux/3 -> Mux1/3
  Demux/2 -> Mux1/2
  Demux/1 -> Mux1/1
  Mux1/1 -> Out1/1
  Mux4/1 -> Out2/1
  Mux3/1 -> Out3/1
  Mux2/1 -> Out4/1

== system nominal_system/(F17-19)(F20-21)(F22)(FF18_FF20_FF22) |X1-22 Chassis Subsystem /(F20_21)(FF20)|X1_22 /Atomic Subsystem1 ==
  In1 : Inport
  Demux : Demux  Outputs=16
  Mux{1..4} (4 alike) : Mux
  Out1 : Outport
  Out2 : Outport  Port=2
  Out3 : Outport  Port=3
  Out4 : Outport  Port=4
  wires:
  In1/1 -> Demux/1
  Demux/16 -> Mux2/4
  Demux/15 -> Mux2/3
  Demux/14 -> Mux2/2
  Demux/13 -> Mux2/1
  Demux/12 -> Mux3/4
  Demux/11 -> Mux3/3
  Demux/10 -> Mux3/2
  Demux/9 -> Mux3/1
  Demux/8 -> Mux4/4
  Demux/7 -> Mux4/3
  Demux/6 -> Mux4/2
  Demux/5 -> Mux4/1
  Demux/4 -> Mux1/4
  Demux/3 -> Mux1/3
  Demux/2 -> Mux1/2
  Demux/1 -> Mux1/1
  Mux1/1 -> Out1/1
  Mux4/1 -> Out2/1
  Mux3/1 -> Out3/1
  Mux2/1 -> Out4/1

== system nominal_system/(F17-19)(F20-21)(F22)(FF18_FF20_FF22) |X1-22 Chassis Subsystem /(F22)(FF22)|X1_22/Atomic Subsystem1 ==
  In1 : Inport
  Demux : Demux  Outputs=16
  Mux{1..4} (4 alike) : Mux
  Out1 : Outport
  Out2 : Outport  Port=2
  Out3 : Outport  Port=3
  Out4 : Outport  Port=4
  wires:
  In1/1 -> Demux/1
  Demux/16 -> Mux2/4
  Demux/15 -> Mux2/3
  Demux/14 -> Mux2/2
  Demux/13 -> Mux2/1
  Demux/12 -> Mux3/4
  Demux/11 -> Mux3/3
  Demux/10 -> Mux3/2
  Demux/9 -> Mux3/1
  Demux/8 -> Mux4/4
  Demux/7 -> Mux4/3
  Demux/6 -> Mux4/2
  Demux/5 -> Mux4/1
  Demux/4 -> Mux1/4
  Demux/3 -> Mux1/3
  Demux/2 -> Mux1/2
  Demux/1 -> Mux1/1
  Mux1/1 -> Out1/1
  Mux4/1 -> Out2/1
  Mux3/1 -> Out3/1
  Mux2/1 -> Out4/1
